simulink model "cartPend_HAC"  (R2023b)
settings: Solver=ode4  StartTime=0.0  StopTime=8  FixedStep=0.001  RelTol=1e-3
values from neighbouring files (symbols this model uses):
  alpha = 5/180*pi    (= 0.0872664625997)    [init_HAC_simulation.m]    (also in my_HAC_improved.m = params.alpha)
  beta = 50/180*pi    (= 0.872664625997)    [init_HAC_simulation.m]    (also in my_HAC_improved.m = params.beta)
  caseSwitch = 2    [init_HAC_simulation.m]
  E_up = m*g*L*cos(0)    [init_HAC_simulation.m]
  eta = 1.3    [init_HAC_simulation.m]
  Fc = 0.00040    (= 0.0004)    [init_HAC_simulation.m]
  g = 9.80665    [init_HAC_simulation.m]
  I = (1/3)*m*L^2    (= 0.0008739525)    [init_HAC_simulation.m]
  init_cont = [x_real(1),xd_real(1),q_real(1),qd_real(1)]    [RSHAC_real_data_processing.m]    (also in init_HAC_simulation.m = [0.1041, -0.2018, deg2rad(-14.9877), deg2rad(135.7108)])
  k_cw = 6    [init_HAC_simulation.m]
  k_em = 10    [init_HAC_simulation.m]
  k_lqr = discrete_lqr(m, M, L, I, g, kd, kt, Fc)    [init_HAC_simulation.m]
  k_su = 2    [init_HAC_simulation.m]
  k_vw = 2.5    [init_HAC_simulation.m]
  kd = 0.000161    [init_HAC_simulation.m]
  kdr = 0.000001    (= 1e-06)    [init_HAC_simulation.m]
  kt = 150    [init_HAC_simulation.m]
  L = 0.3/2    (= 0.15)    [init_HAC_simulation.m]
  m = 0.116527    [init_HAC_simulation.m]
  q_max = deg2rad(20)    [init_HAC_simulation.m]    (also in my_HAC_improved.m = X_max(3))
  q_min = -q_max    (= -0.261799387799)    [init_HAC_simulation.m]    (also in my_HAC_improved.m = X_min(3))
  q_sqm = zeros(1, n_rules_q)    [init_HAC_simulation.m]
  qd_max = 6    [init_HAC_simulation.m]    (also in my_HAC_improved.m = X_max(4))
  qd_min = -qd_max    (= -6)    [init_HAC_simulation.m]    (also in my_HAC_improved.m = X_min(4))
  qd_sqm = zeros(1, n_rules_qd)    [init_HAC_simulation.m]
  SQMs_state = zeros(1,n_rules)    [init_HAC_simulation.m]
  SQMs_u = zeros(1,n_rules)    [init_HAC_simulation.m]
  target_pos = 0    [init_HAC_simulation.m]
  u_max = 3 * g    (= 29.41995)    [init_HAC_simulation.m]    (also in my_HAC_improved.m = params.u_max)
  u_min = -u_max    (= -29.41995)    [init_HAC_simulation.m]    (also in my_HAC_improved.m = params.u_min)
  u_q_sqm = zeros(1, n_rules_q)    [init_HAC_simulation.m]
  u_qd_sqm = zeros(1, n_rules_qd)    [init_HAC_simulation.m]
  u_x_sqm = zeros(1, n_rules_x)    [init_HAC_simulation.m]
  u_xd_sqm = zeros(1, n_rules_xd)    [init_HAC_simulation.m]
  uMax = 3*g    (= 29.41995)    [init_HAC_simulation.m]
  w_high = 1    [init_HAC_simulation.m]    (also in my_HAC_improved.m = params.w_high)
  w_low = 0.25    [init_HAC_simulation.m]    (also in my_HAC_improved.m = params.w_low)
  x1_max = 0.43    [init_HAC_simulation.m]
  x2_max = 2    [init_HAC_simulation.m]
  x_max = 0.43    [init_HAC_simulation.m]    (also in my_HAC_improved.m = X_max(1))
  x_min = -x_max    (= -0.43)    [init_HAC_simulation.m]    (also in my_HAC_improved.m = X_min(1))
  x_sqm = zeros(1, n_rules_x)    [init_HAC_simulation.m]
  xd_max = 2.0    (= 2)    [init_HAC_simulation.m]    (also in my_HAC_improved.m = X_max(2))
  xd_min = -xd_max    (= -2)    [init_HAC_simulation.m]    (also in my_HAC_improved.m = X_min(2))
  xd_sqm = zeros(1, n_rules_xd)    [init_HAC_simulation.m]
undefined symbols (not defined in the file or in its folder): useThayLe
libraries: fuzblock x7, simulink x5, simulink_extras x2
settings Model: Creator=doann  LastModifiedBy=doann
settings OptimizationCC: ReuseModelBlockBuffer=off

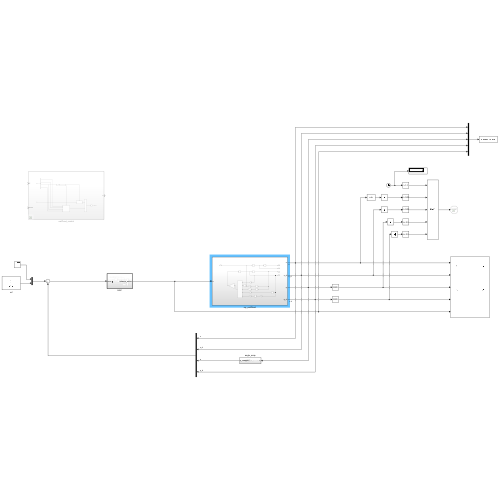
[thumbnail: Simulink's stored preview of the top-level diagram]
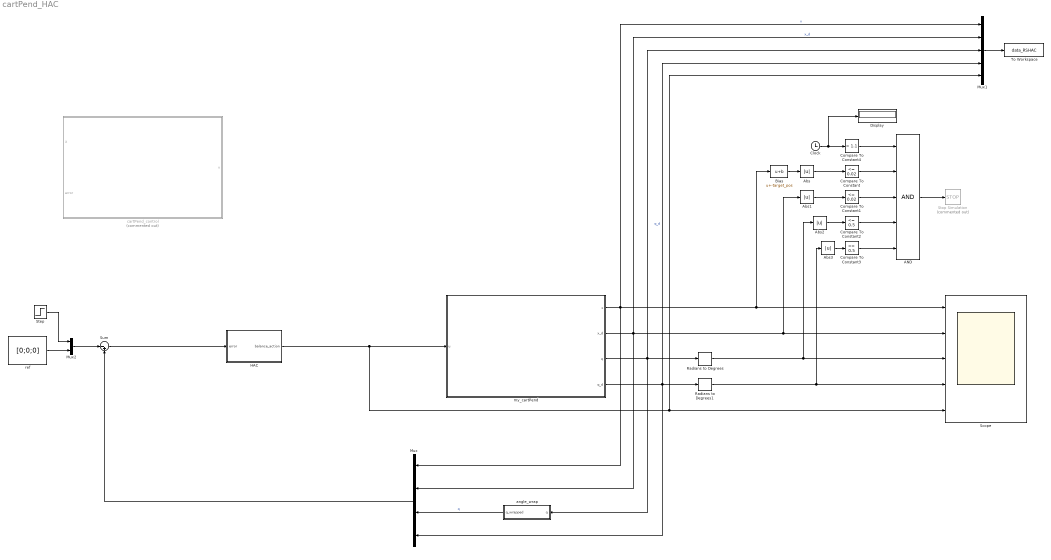
== system cartPend_HAC ==
  AND : Logic  Inputs=5  AllPortsSameDT=off  OutDataTypeStr=boolean
  Abs{,1..3} (4 alike) : Abs  SaturateOnIntegerOverflow=off
  Bias : Bias  Bias=-target_pos  SaturateOnIntegerOverflow=off
  Clock : Clock
  Compare To Constant : simulink/Logic and Bit Operations/Compare To Constant  relop=<=  const=0.02  OutDataTypeStr=boolean
  Compare To Constant1 : simulink/Logic and Bit Operations/Compare To Constant  relop=<=  const=0.02  OutDataTypeStr=boolean
  Compare To Constant2 : simulink/Logic and Bit Operations/Compare To Constant  relop=<=  const=0.5  OutDataTypeStr=boolean
  Compare To Constant3 : simulink/Logic and Bit Operations/Compare To Constant  relop=<=  const=0.5  OutDataTypeStr=boolean
  Compare To Constant4 : simulink/Logic and Bit Operations/Compare To Constant  relop=>  const=1.1  OutDataTypeStr=boolean
  Display : Display
  HAC : Subsystem  TreatAsAtomicUnit=on
  Mux : Mux
  Mux1 : Mux  Inputs=5
  Mux2 : Mux  Inputs=2
  Radians to Degrees : simulink_extras/Transformations/Radians to Degrees
  Radians to Degrees1 : simulink_extras/Transformations/Radians to Degrees
  Scope : Scope  NumInputPorts=5
  Step : Step  After=target_pos  SampleTime=0
  Stop Simulation : Stop  Commented=on
  Sum : Sum  Inputs=|-+
  To Workspace : ToWorkspace  VariableName=data_RSHAC  SaveFormat=Timeseries  SampleTime=-1
  angle_wrap : Subsystem
  cartPend_control : Subsystem  Commented=on  SystemSampleTime=0.001
  my_cartPend : Subsystem
  ref : Constant  Value=[0;0;0]  VectorParams1D=off
  wires:
  my_cartPend/1(x) -> Mux1/1, Bias/1, Scope/1, Mux/1  "x"
  my_cartPend/2(x_d) -> Mux1/2, Abs1/1, Scope/2, Mux/2  "x_d"
  Radians to Degrees/1 -> Abs2/1, Scope/3
  my_cartPend/4(q_d) -> Mux1/4, Radians to Degrees1/1, Mux/4  "q_d"
  Radians to Degrees1/1 -> Abs3/1, Scope/4
  my_cartPend/3(q) -> Mux1/3, Radians to Degrees/1, angle_wrap/1(q)
  angle_wrap/1(q_wrapped) -> Mux/3  "q"
  Mux/1 -> Sum/2
  Mux1/1 -> To Workspace/1
  Sum/1 -> HAC/1(error)
  HAC/1(balance_action) -> Mux1/5, Scope/5, my_cartPend/1(u)
  Compare To Constant/1 -> AND/2
  Compare To Constant1/1 -> AND/3
  Compare To Constant2/1 -> AND/4
  Compare To Constant3/1 -> AND/5
  Abs/1 -> Compare To Constant/1
  Abs1/1 -> Compare To Constant1/1
  Abs2/1 -> Compare To Constant2/1
  Abs3/1 -> Compare To Constant3/1
  Clock/1 -> Display/1, Compare To Constant4/1
  Compare To Constant4/1 -> AND/1
  Bias/1 -> Abs/1
  Step/1 -> Mux2/1
  ref/1 -> Mux2/2
  Mux2/1 -> Sum/1
  AND/1 -> Stop Simulation/1

== system cartPend_HAC/HAC ==
  error : Inport
  Constant : Constant  Value=caseSwitch
  Fuzzy_controller : Subsystem  TreatAsAtomicUnit=on
  HAC_thay_Le : Subsystem
  LQR : Subsystem
  Merge : Merge  Inputs=4
  RSHAC : Subsystem
  Switch Case : SwitchCase  CaseConditions={1,2,3,4}  ShowDefaultCase=off
  balance_action : Outport
  wires:
  error/1 -> HAC_thay_Le/1(error), RSHAC/1(error), Fuzzy_controller/1(error), LQR/1(error)
  Constant/1 -> Switch Case/1
  Switch Case/3 -> HAC_thay_Le/Action
  Switch Case/2 -> RSHAC/Action
  Switch Case/1 -> LQR/Action
  HAC_thay_Le/1(u) -> Merge/1
  RSHAC/1(u) -> Merge/2
  LQR/1(u) -> Merge/3
  Merge/1 -> balance_action/1
  Fuzzy_controller/1(u) -> Merge/4
  Switch Case/4 -> Fuzzy_controller/Action

== system cartPend_HAC/angle_wrap ==
  q : Inport
  Atan2 : Trigonometry  Operator=atan2
  Cos : Trigonometry  Operator=cos
  Sin : Trigonometry
  q_wrapped : Outport
  wires:
  Atan2/1 -> q_wrapped/1
  Sin/1 -> Atan2/1
  q/1 -> Cos/1, Sin/1
  Cos/1 -> Atan2/2

== system cartPend_HAC/cartPend_control ==
  X : Inport
  error : Inport  Port=2
  Abs : Abs  SaturateOnIntegerOverflow=off
  Demux : Demux
  HAC : Subsystem  TreatAsAtomicUnit=on
  If : If  IfExpression=u1 < angle_threshold
  Merge : Merge
  Saturation : Saturate  UpperLimit=uMax  LowerLimit=-uMax
  energy swing up : Subsystem  TreatAsAtomicUnit=on
  u : Outport
  wires:
  X/1 -> Demux/1
  Demux/3 -> Abs/1, energy swing up/3(x3)  "x3"
  Demux/4 -> energy swing up/4(x4)  "x4"
  Abs/1 -> If/1
  If/1 -> HAC/Action
  If/2 -> energy swing up/Action
  HAC/1(balance_action) -> Merge/1
  energy swing up/1(swing_up_action) -> Merge/2
  error/1 -> HAC/1(error)
  Demux/2 -> energy swing up/2(x2)  "x2"
  Demux/1 -> energy swing up/1(x1)  "x1"
  Merge/1 -> Saturation/1
  Saturation/1 -> u/1

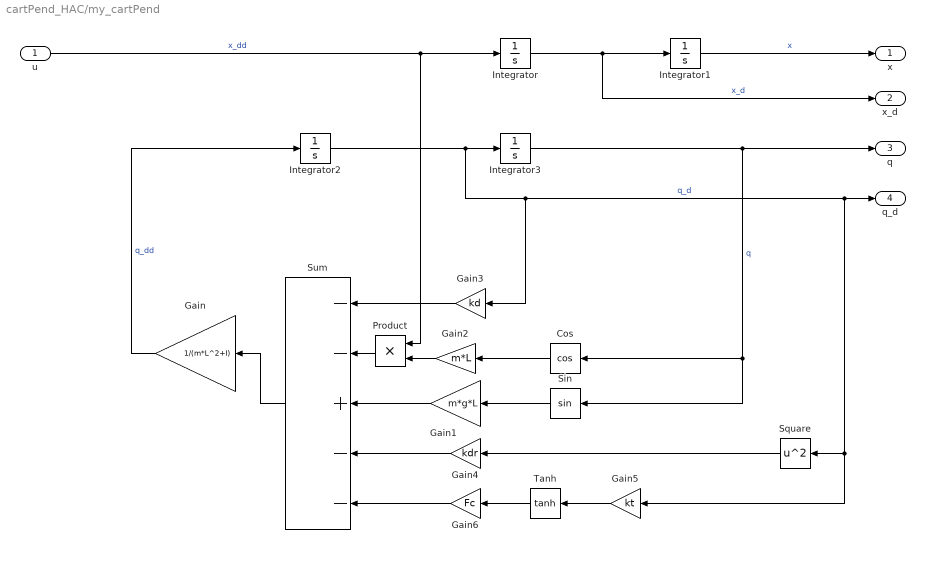
== system cartPend_HAC/my_cartPend ==
  u : Inport
  Cos : Trigonometry  Operator=cos
  Gain : Gain  Gain=1/(m*L^2+I)
  Gain1 : Gain  Gain=m*g*L
  Gain2 : Gain  Gain=m*L
  Gain3 : Gain  Gain=kd
  Gain4 : Gain  Gain=kdr
  Gain5 : Gain  Gain=kt
  Gain6 : Gain  Gain=Fc
  Integrator : Integrator  InitialCondition=init_cont(2)
  Integrator1 : Integrator  InitialCondition=init_cont(1)
  Integrator2 : Integrator  InitialCondition=init_cont(4)
  Integrator3 : Integrator  InitialCondition=init_cont(3)
  Product : Product
  Sin : Trigonometry
  Square : Math  Operator=square
  Sum : Sum  Inputs=--+--
  Tanh : Trigonometry  Operator=tanh
  x : Outport
  x_d : Outport  Port=2
  q : Outport  Port=3
  q_d : Outport  Port=4
  wires:
  Gain6/1 -> Sum/5
  Gain4/1 -> Sum/4
  Gain5/1 -> Tanh/1
  Tanh/1 -> Gain6/1
  Square/1 -> Gain4/1
  Product/1 -> Sum/2
  Gain2/1 -> Product/2
  Gain3/1 -> Sum/1
  Gain1/1 -> Sum/3
  Gain/1 -> Integrator2/1  "q_dd"
  Sum/1 -> Gain/1
  Cos/1 -> Gain2/1
  Sin/1 -> Gain1/1
  Integrator2/1 -> Integrator3/1, q_d/1, Square/1, Gain5/1, Gain3/1  "q_d"
  Integrator3/1 -> q/1, Cos/1, Sin/1  "q"
  Integrator1/1 -> x/1  "x"
  Integrator/1 -> Integrator1/1, x_d/1  "x_d"
  u/1 -> Integrator/1, Product/1  "x_dd"

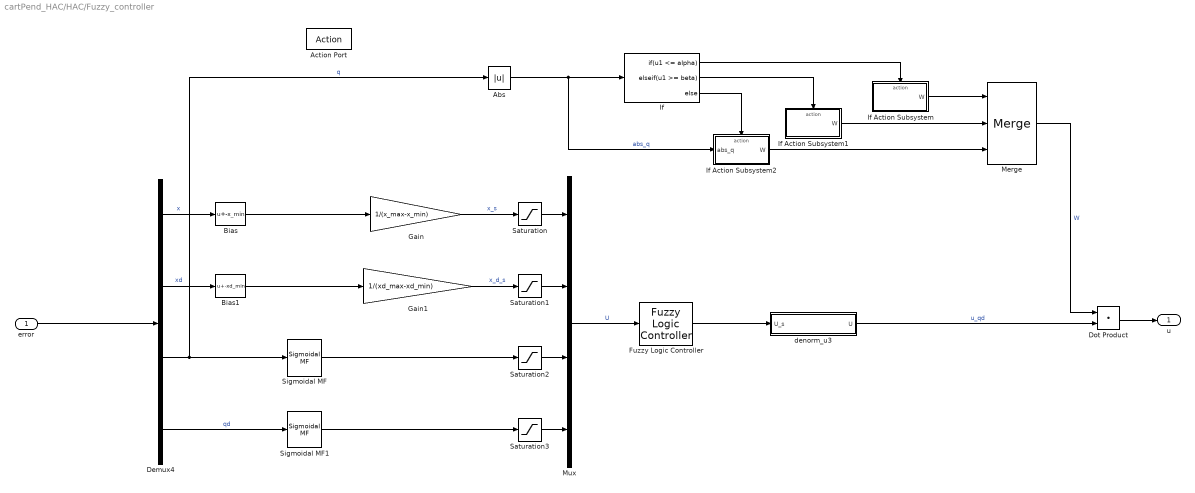
== system cartPend_HAC/HAC/Fuzzy_controller ==
  error : Inport
  Action Port : ActionPort  ActionPortLabel=case [ 4 ]:
  Abs : Abs  SaturateOnIntegerOverflow=off
  Bias : Bias  Bias=-x_min  SaturateOnIntegerOverflow=off
  Bias1 : Bias  Bias=-xd_min  SaturateOnIntegerOverflow=off
  Demux4 : Demux
  Dot Product : DotProduct  OutDataTypeStr=Inherit: Inherit via internal rule
  Fuzzy Logic Controller : fuzblock/Fuzzy Logic  Controller  FIS='fuzzy_ctrl_v2.fis'  OutputSampleNumber=101  DataType=double  FuzzifiedInputs=off  RuleFiringStrengths=off  RuleOutputs=off  AggregatedOutputs=off  SimulateUsing=Interpreted execution  OutOfRangeInputValueMessage=warning  NoRuleFiredMessage=warning  EmptyOutputFuzzySetMessage=warning
  Gain : Gain  Gain=1/(x_max-x_min)
  Gain1 : Gain  Gain=1/(xd_max-xd_min)
  If : If  IfExpression=u1 <= alpha  ElseIfExpressions=u1 >= beta
  If Action Subsystem : Subsystem  TreatAsAtomicUnit=on
  If Action Subsystem1 : Subsystem  TreatAsAtomicUnit=on
  If Action Subsystem2 : Subsystem  TreatAsAtomicUnit=on
  Merge : Merge  Inputs=3
  Mux : Mux
  Saturation{,1..3} (4 alike) : Saturate  UpperLimit=0.75  LowerLimit=0.25
  Sigmoidal MF : fuzblock/Membership  Functions/Sigmoidal MF  a=a_sigmoid_q  c=0
  Sigmoidal MF1 : fuzblock/Membership  Functions/Sigmoidal MF  a=a_sigmoid_q_d  c=0
  denorm_u3 : Subsystem
  u : Outport
  wires:
  Demux4/2 -> Bias1/1  "xd"
  Gain/1 -> Saturation/1  "x_s"
  Sigmoidal MF/1 -> Saturation2/1
  Demux4/4 -> Sigmoidal MF1/1  "qd"
  Bias/1 -> Gain/1
  Gain1/1 -> Saturation1/1  "x_d_s"
  Sigmoidal MF1/1 -> Saturation3/1
  Bias1/1 -> Gain1/1
  Demux4/1 -> Bias/1  "x"
  error/1 -> Demux4/1
  Mux/1 -> Fuzzy Logic Controller/1  "U"
  Fuzzy Logic Controller/1 -> denorm_u3/1(U_s)
  Saturation/1 -> Mux/1
  Saturation1/1 -> Mux/2
  Saturation2/1 -> Mux/3
  Saturation3/1 -> Mux/4
  If/2 -> If Action Subsystem1/Action
  If Action Subsystem2/1(W) -> Merge/3
  If/1 -> If Action Subsystem/Action
  If Action Subsystem1/1(W) -> Merge/2
  If/3 -> If Action Subsystem2/Action
  Demux4/3 -> Sigmoidal MF/1, Abs/1  "q"
  Abs/1 -> If Action Subsystem2/1(abs_q), If/1  "abs_q"
  If Action Subsystem/1(W) -> Merge/1
  Merge/1 -> Dot Product/1  "W"
  denorm_u3/1(U) -> Dot Product/2  "u_qd"
  Dot Product/1 -> u/1

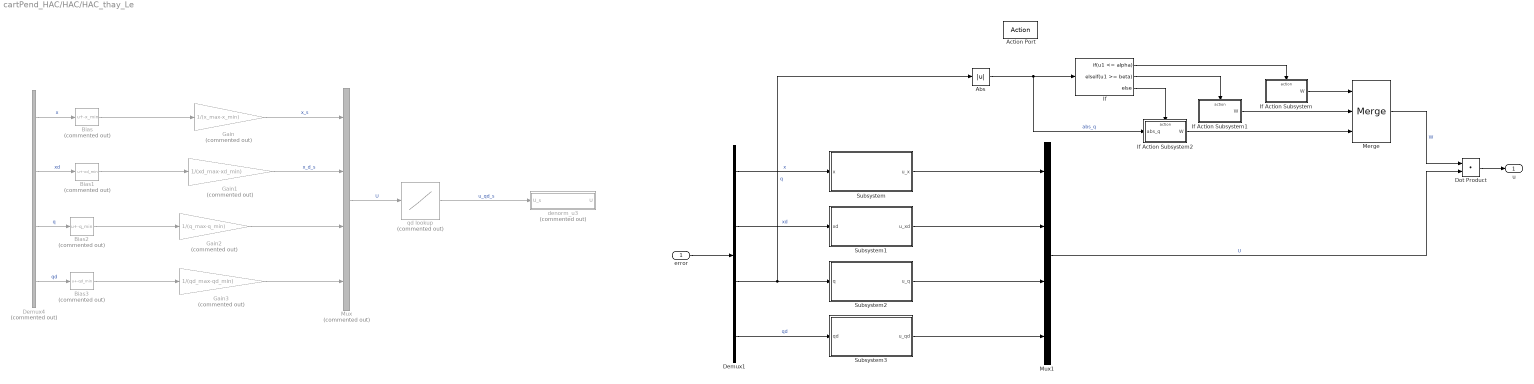
== system cartPend_HAC/HAC/HAC_thay_Le ==
  error : Inport
  Action Port : ActionPort  ActionPortLabel=case [ 3 ]:
  Abs : Abs  SaturateOnIntegerOverflow=off
  Bias : Bias  Commented=on  Bias=-x_min  SaturateOnIntegerOverflow=off
  Bias1 : Bias  Commented=on  Bias=-xd_min  SaturateOnIntegerOverflow=off
  Bias2 : Bias  Commented=on  Bias=-q_min  SaturateOnIntegerOverflow=off
  Bias3 : Bias  Commented=on  Bias=-qd_min  SaturateOnIntegerOverflow=off
  Demux1 : Demux
  Demux4 : Demux  Commented=on
  Dot Product : DotProduct  OutDataTypeStr=Inherit: Inherit via internal rule
  Gain : Gain  Commented=on  Gain=1/(x_max-x_min)
  Gain1 : Gain  Commented=on  Gain=1/(xd_max-xd_min)
  Gain2 : Gain  Commented=on  Gain=1/(q_max-q_min)
  Gain3 : Gain  Commented=on  Gain=1/(qd_max-qd_min)
  If : If  IfExpression=u1 <= alpha  ElseIfExpressions=u1 >= beta
  If Action Subsystem : Subsystem  TreatAsAtomicUnit=on
  If Action Subsystem1 : Subsystem  TreatAsAtomicUnit=on
  If Action Subsystem2 : Subsystem  TreatAsAtomicUnit=on
  Merge : Merge  Inputs=3
  Mux : Mux  Commented=on
  Mux1 : Mux
  Subsystem : Subsystem
  Subsystem1 : Subsystem
  Subsystem2 : Subsystem
  Subsystem3 : Subsystem
  denorm_u3 : Subsystem  Commented=on
  qd lookup : Lookup_n-D  Commented=on  NumberOfTableDimensions=1  BreakpointsForDimension1=SQMs_state  Table=SQMs_u  InternalRulePriority=Speed  RndMeth=Simplest
  u : Outport
  wires:
  Merge/1 -> Dot Product/1  "W"
  Demux4/4 -> Bias3/1  "qd"
  qd lookup/1 -> denorm_u3/1(U_s)  "u_qd_s"
  Bias3/1 -> Gain3/1
  Bias2/1 -> Gain2/1
  Demux4/2 -> Bias1/1  "xd"
  Bias1/1 -> Gain1/1
  Demux4/1 -> Bias/1  "x"
  Bias/1 -> Gain/1
  Dot Product/1 -> u/1
  If Action Subsystem2/1(W) -> Merge/3
  If Action Subsystem1/1(W) -> Merge/2
  If Action Subsystem/1(W) -> Merge/1
  If/3 -> If Action Subsystem2/Action
  If/2 -> If Action Subsystem1/Action
  If/1 -> If Action Subsystem/Action
  Abs/1 -> If Action Subsystem2/1(abs_q), If/1  "abs_q"
  Demux4/3 -> Bias2/1  "q"
  Gain1/1 -> Mux/2  "x_d_s"
  Gain/1 -> Mux/1  "x_s"
  Gain2/1 -> Mux/3
  Gain3/1 -> Mux/4
  Mux/1 -> qd lookup/1  "U"
  Demux1/1 -> Subsystem/1(x)  "x"
  Subsystem/1(u_x) -> Mux1/1
  Demux1/2 -> Subsystem1/1(xd)  "xd"
  Subsystem1/1(u_xd) -> Mux1/2
  Demux1/3 -> Abs/1, Subsystem2/1(q)  "q"
  Subsystem2/1(u_q) -> Mux1/3
  Demux1/4 -> Subsystem3/1(qd)  "qd"
  Subsystem3/1(u_qd) -> Mux1/4
  error/1 -> Demux1/1
  Mux1/1 -> Dot Product/2  "U"

== system cartPend_HAC/HAC/LQR ==
  error : Inport
  Action Port : ActionPort  ActionPortLabel=case [ 1 ]:
  Gain : Gain  Gain=k_lqr  Multiplication=Matrix(K*u)
  Gain1 : Gain  Gain=-1
  u : Outport
  wires:
  Gain1/1 -> Gain/1
  Gain/1 -> u/1
  error/1 -> Gain1/1

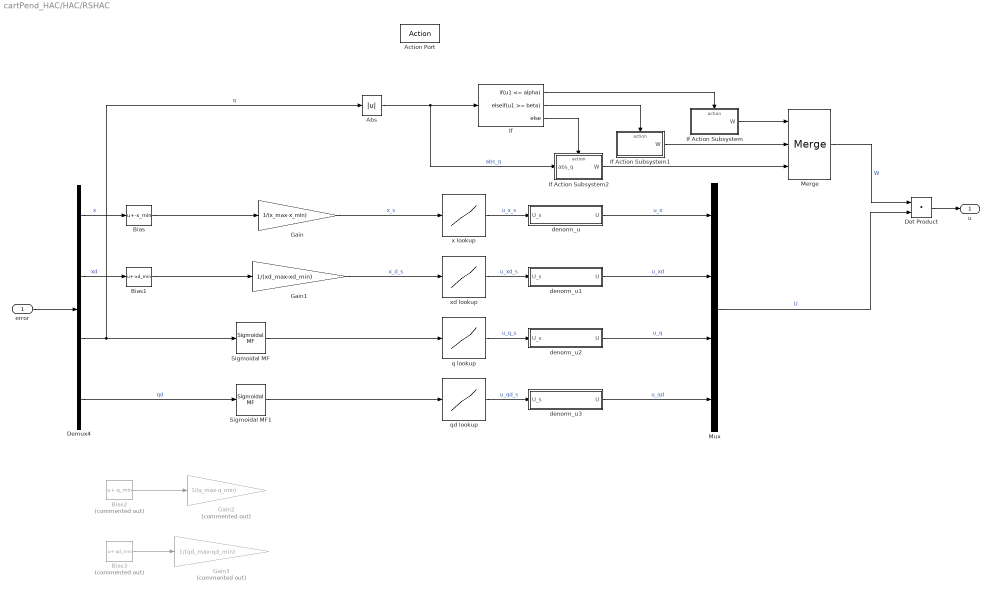
== system cartPend_HAC/HAC/RSHAC ==
  error : Inport
  Action Port : ActionPort  ActionPortLabel=case [ 2 ]:
  Abs : Abs  SaturateOnIntegerOverflow=off
  Bias : Bias  Bias=-x_min  SaturateOnIntegerOverflow=off
  Bias1 : Bias  Bias=-xd_min  SaturateOnIntegerOverflow=off
  Bias2 : Bias  Commented=on  Bias=-q_min  SaturateOnIntegerOverflow=off
  Bias3 : Bias  Commented=on  Bias=-qd_min  SaturateOnIntegerOverflow=off
  Demux4 : Demux
  Dot Product : DotProduct  OutDataTypeStr=Inherit: Inherit via internal rule
  Gain : Gain  Gain=1/(x_max-x_min)
  Gain1 : Gain  Gain=1/(xd_max-xd_min)
  Gain2 : Gain  Commented=on  Gain=1/(q_max-q_min)
  Gain3 : Gain  Commented=on  Gain=1/(qd_max-qd_min)
  If : If  IfExpression=u1 <= alpha  ElseIfExpressions=u1 >= beta
  If Action Subsystem : Subsystem  TreatAsAtomicUnit=on
  If Action Subsystem1 : Subsystem  TreatAsAtomicUnit=on
  If Action Subsystem2 : Subsystem  TreatAsAtomicUnit=on
  Merge : Merge  Inputs=3
  Mux : Mux
  Sigmoidal MF : fuzblock/Membership  Functions/Sigmoidal MF  a=a_sigmoid_q  c=0
  Sigmoidal MF1 : fuzblock/Membership  Functions/Sigmoidal MF  a=a_sigmoid_q_d  c=0
  denorm_u : Subsystem
  denorm_u1 : Subsystem
  denorm_u2 : Subsystem
  denorm_u3 : Subsystem
  q lookup : Lookup_n-D  NumberOfTableDimensions=1  BreakpointsForDimension1=q_sqm  Table=u_q_sqm  InternalRulePriority=Speed  RndMeth=Simplest
  qd lookup : Lookup_n-D  NumberOfTableDimensions=1  BreakpointsForDimension1=qd_sqm  Table=u_qd_sqm  InternalRulePriority=Speed  RndMeth=Simplest
  x lookup : Lookup_n-D  NumberOfTableDimensions=1  BreakpointsForDimension1=x_sqm  Table=u_x_sqm  InternalRulePriority=Speed  RndMeth=Simplest
  xd lookup : Lookup_n-D  NumberOfTableDimensions=1  BreakpointsForDimension1=xd_sqm  Table=u_xd_sqm  InternalRulePriority=Speed  RndMeth=Simplest
  u : Outport
  wires:
  Demux4/3 -> Sigmoidal MF/1, Abs/1  "q"
  Gain/1 -> x lookup/1  "x_s"
  Abs/1 -> If Action Subsystem2/1(abs_q), If/1  "abs_q"
  If/1 -> If Action Subsystem/Action
  If/2 -> If Action Subsystem1/Action
  If/3 -> If Action Subsystem2/Action
  If Action Subsystem/1(W) -> Merge/1
  If Action Subsystem1/1(W) -> Merge/2
  If Action Subsystem2/1(W) -> Merge/3
  Dot Product/1 -> u/1
  error/1 -> Demux4/1
  Bias/1 -> Gain/1
  Demux4/1 -> Bias/1  "x"
  Bias1/1 -> Gain1/1
  Gain1/1 -> xd lookup/1  "x_d_s"
  Demux4/2 -> Bias1/1  "xd"
  Bias2/1 -> Gain2/1
  Bias3/1 -> Gain3/1
  x lookup/1 -> denorm_u/1(U_s)  "u_x_s"
  denorm_u/1(U) -> Mux/1  "u_x"
  xd lookup/1 -> denorm_u1/1(U_s)  "u_xd_s"
  denorm_u1/1(U) -> Mux/2  "u_xd"
  q lookup/1 -> denorm_u2/1(U_s)  "u_q_s"
  denorm_u2/1(U) -> Mux/3  "u_q"
  qd lookup/1 -> denorm_u3/1(U_s)  "u_qd_s"
  denorm_u3/1(U) -> Mux/4  "u_qd"
  Mux/1 -> Dot Product/2  "U"
  Sigmoidal MF/1 -> q lookup/1
  Sigmoidal MF1/1 -> qd lookup/1
  Demux4/4 -> Sigmoidal MF1/1  "qd"
  Merge/1 -> Dot Product/1  "W"

== system cartPend_HAC/cartPend_control/HAC ==
  error : Inport
  Action Port : ActionPort  ActionPortLabel=if(u1 < angle_threshold)
  Constant : Constant  Value=useThayLe
  HAC : Subsystem
  HAC_thay_Le : Subsystem
  Switch : Switch  Criteria=u2 ~= 0  SaturateOnIntegerOverflow=off  InputSameDT=off
  balance_action : Outport
  wires:
  Constant/1 -> Switch/2
  HAC_thay_Le/1(u) -> Switch/1
  HAC/1(u) -> Switch/3
  Switch/1 -> balance_action/1
  error/1 -> HAC/1(error), HAC_thay_Le/1(error)

== system cartPend_HAC/cartPend_control/energy swing up ==
  x1 : Inport
  x2 : Inport  Port=2
  x3 : Inport  Port=3
  x4 : Inport  Port=4
  Action Port : ActionPort  ActionPortLabel=else
  Sum : Sum  Inputs=++++
  energy injection : Subsystem
  energy maintenance : Subsystem
  position potential well : Subsystem
  velocity potential well : Subsystem
  swing_up_action : Outport
  wires:
  energy injection/1(u_su) -> Sum/3
  x2/1 -> velocity potential well/1(x2)  "x2"
  velocity potential well/1(u_vw) -> Sum/2
  Sum/1 -> swing_up_action/1
  energy maintenance/1(u_em) -> Sum/4
  x3/1 -> energy maintenance/1(x3), energy injection/1(x3)  "x3"
  x1/1 -> position potential well/1(x1)  "x1"
  x4/1 -> energy injection/2(x4), energy maintenance/2(x4)  "x4"
  position potential well/1(u_cw) -> Sum/1

== system cartPend_HAC/HAC/Fuzzy_controller/If Action Subsystem ==
  Action Port : ActionPort  ActionPortLabel=if(u1 <= alpha)
  weight : Constant  Value=[0.25; 0.25; 0.25; 0.25]  VectorParams1D=off
  W : Outport
  wires:
  weight/1 -> W/1

== system cartPend_HAC/HAC/Fuzzy_controller/If Action Subsystem1 ==
  Action Port : ActionPort  ActionPortLabel=elseif(u1 >= beta)
  weights : Constant  Value=[0; 0; 1; 0]  VectorParams1D=off
  W : Outport
  wires:
  weights/1 -> W/1

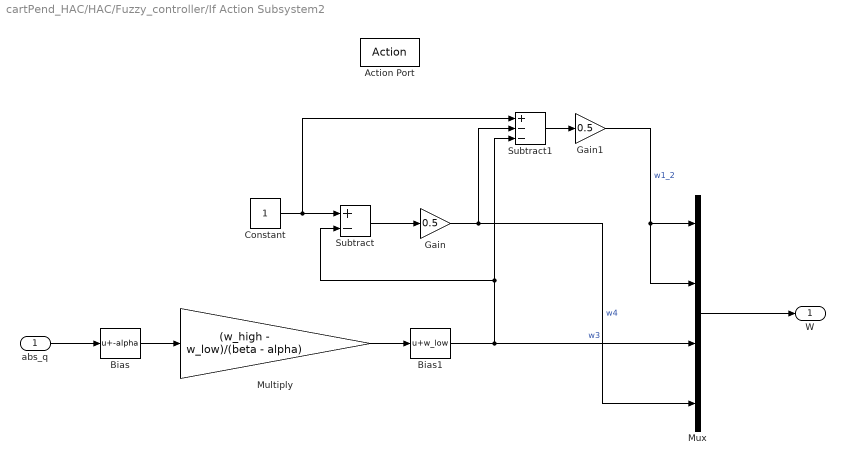
== system cartPend_HAC/HAC/Fuzzy_controller/If Action Subsystem2 ==
  abs_q : Inport
  Action Port : ActionPort  ActionPortLabel=else
  Bias : Bias  Bias=-alpha  SaturateOnIntegerOverflow=off
  Bias1 : Bias  Bias=w_low  SaturateOnIntegerOverflow=off
  Constant : Constant
  Gain : Gain  Gain=0.5
  Gain1 : Gain  Gain=0.5
  Multiply : Gain  Gain=(w_high - w_low)/(beta - alpha)
  Mux : Mux
  Subtract : Sum  Inputs=+-
  Subtract1 : Sum  Inputs=+--
  W : Outport
  wires:
  Mux/1 -> W/1
  abs_q/1 -> Bias/1
  Bias/1 -> Multiply/1
  Multiply/1 -> Bias1/1
  Bias1/1 -> Subtract/2, Subtract1/3, Mux/3  "w3"
  Constant/1 -> Subtract1/1, Subtract/1
  Subtract/1 -> Gain/1
  Gain/1 -> Subtract1/2, Mux/4  "w4"
  Subtract1/1 -> Gain1/1
  Gain1/1 -> Mux/1, Mux/2  "w1_2"

== system cartPend_HAC/HAC/Fuzzy_controller/denorm_u3 ==
  U_s : Inport
  Bias : Bias  Bias=2*u_min  SaturateOnIntegerOverflow=off
  Gain : Gain  Gain=4*u_max
  U : Outport
  wires:
  U_s/1 -> Gain/1
  Gain/1 -> Bias/1
  Bias/1 -> U/1

== system cartPend_HAC/HAC/HAC_thay_Le/If Action Subsystem ==
  Action Port : ActionPort  ActionPortLabel=if(u1 <= alpha)
  weight : Constant  Value=[0.25; 0.25; 0.25; 0.25]  VectorParams1D=off
  W : Outport
  wires:
  weight/1 -> W/1

== system cartPend_HAC/HAC/HAC_thay_Le/If Action Subsystem1 ==
  Action Port : ActionPort  ActionPortLabel=elseif(u1 >= beta)
  weights : Constant  Value=[0; 0; 1; 0]  VectorParams1D=off
  W : Outport
  wires:
  weights/1 -> W/1

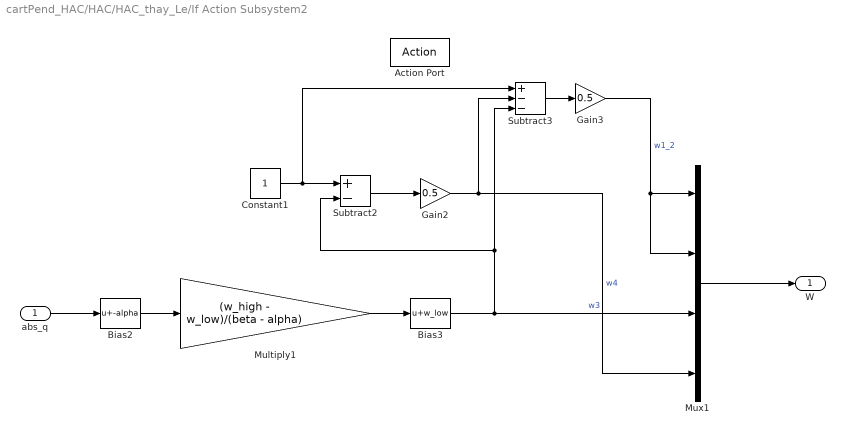
== system cartPend_HAC/HAC/HAC_thay_Le/If Action Subsystem2 ==
  abs_q : Inport
  Action Port : ActionPort  ActionPortLabel=else
  Bias2 : Bias  Bias=-alpha  SaturateOnIntegerOverflow=off
  Bias3 : Bias  Bias=w_low  SaturateOnIntegerOverflow=off
  Constant1 : Constant
  Gain2 : Gain  Gain=0.5
  Gain3 : Gain  Gain=0.5
  Multiply1 : Gain  Gain=(w_high - w_low)/(beta - alpha)
  Mux1 : Mux
  Subtract2 : Sum  Inputs=+-
  Subtract3 : Sum  Inputs=+--
  W : Outport
  wires:
  Subtract3/1 -> Gain3/1
  Gain2/1 -> Subtract3/2, Mux1/4  "w4"
  Bias3/1 -> Subtract2/2, Subtract3/3, Mux1/3  "w3"
  Bias2/1 -> Multiply1/1
  Gain3/1 -> Mux1/1, Mux1/2  "w1_2"
  Subtract2/1 -> Gain2/1
  Multiply1/1 -> Bias3/1
  Constant1/1 -> Subtract3/1, Subtract2/1
  Mux1/1 -> W/1
  abs_q/1 -> Bias2/1

== system cartPend_HAC/HAC/HAC_thay_Le/Subsystem ==
  x : Inport
  If Action Subsystem3 : Subsystem  TreatAsAtomicUnit=on
  If Action Subsystem4 : Subsystem  TreatAsAtomicUnit=on
  If Action Subsystem5 : Subsystem  TreatAsAtomicUnit=on
  If1 : If  IfExpression=u1 <= x_min  ElseIfExpressions=u1 >= x_max
  Merge1 : Merge  Inputs=3
  u_x : Outport
  wires:
  If1/1 -> If Action Subsystem3/Action
  If Action Subsystem3/1(u_min) -> Merge1/1
  Merge1/1 -> u_x/1
  x/1 -> If Action Subsystem5/1(x), If1/1
  If1/3 -> If Action Subsystem5/Action
  If1/2 -> If Action Subsystem4/Action
  If Action Subsystem5/1(u_x) -> Merge1/3
  If Action Subsystem4/1(u_max) -> Merge1/2

== system cartPend_HAC/HAC/HAC_thay_Le/Subsystem1 ==
  xd : Inport
  If Action Subsystem3 : Subsystem  TreatAsAtomicUnit=on
  If Action Subsystem4 : Subsystem  TreatAsAtomicUnit=on
  If Action Subsystem5 : Subsystem  TreatAsAtomicUnit=on
  If1 : If  IfExpression=u1 <= xd_min  ElseIfExpressions=u1 >= xd_max
  Merge1 : Merge  Inputs=3
  u_xd : Outport
  wires:
  If Action Subsystem4/1(u_max) -> Merge1/2
  If Action Subsystem5/1(u_xd) -> Merge1/3
  If1/2 -> If Action Subsystem4/Action
  If1/3 -> If Action Subsystem5/Action
  xd/1 -> If1/1, If Action Subsystem5/1(xd)
  Merge1/1 -> u_xd/1
  If Action Subsystem3/1(u_min) -> Merge1/1
  If1/1 -> If Action Subsystem3/Action

== system cartPend_HAC/HAC/HAC_thay_Le/Subsystem2 ==
  q : Inport
  If Action Subsystem3 : Subsystem  TreatAsAtomicUnit=on
  If Action Subsystem4 : Subsystem  TreatAsAtomicUnit=on
  If Action Subsystem5 : Subsystem  TreatAsAtomicUnit=on
  If1 : If  IfExpression=u1 <= q_min  ElseIfExpressions=u1 >= q_max
  Merge1 : Merge  Inputs=3
  u_q : Outport
  wires:
  If1/1 -> If Action Subsystem3/Action
  If Action Subsystem3/1(u_min) -> Merge1/1
  Merge1/1 -> u_q/1
  q/1 -> If Action Subsystem5/1(q), If1/1
  If1/3 -> If Action Subsystem5/Action
  If1/2 -> If Action Subsystem4/Action
  If Action Subsystem5/1(u_q) -> Merge1/3
  If Action Subsystem4/1(u_max) -> Merge1/2

== system cartPend_HAC/HAC/HAC_thay_Le/Subsystem3 ==
  qd : Inport
  If Action Subsystem3 : Subsystem  TreatAsAtomicUnit=on
  If Action Subsystem4 : Subsystem  TreatAsAtomicUnit=on
  If Action Subsystem5 : Subsystem  TreatAsAtomicUnit=on
  If1 : If  IfExpression=u1 <= qd_min  ElseIfExpressions=u1 >= qd_max
  Merge1 : Merge  Inputs=3
  u_qd : Outport
  wires:
  If Action Subsystem4/1(u_max) -> Merge1/2
  If Action Subsystem5/1(u_qd) -> Merge1/3
  If1/2 -> If Action Subsystem4/Action
  If1/3 -> If Action Subsystem5/Action
  qd/1 -> If1/1, If Action Subsystem5/1(qd)
  Merge1/1 -> u_qd/1
  If Action Subsystem3/1(u_min) -> Merge1/1
  If1/1 -> If Action Subsystem3/Action

== system cartPend_HAC/HAC/HAC_thay_Le/denorm_u3 ==
  U_s : Inport
  Bias : Bias  Bias=u_min  SaturateOnIntegerOverflow=off
  Gain : Gain  Gain=u_max - u_min
  U : Outport
  wires:
  U_s/1 -> Gain/1
  Gain/1 -> Bias/1
  Bias/1 -> U/1

== system cartPend_HAC/HAC/RSHAC/If Action Subsystem ==
  Action Port : ActionPort  ActionPortLabel=if(u1 <= alpha)
  weight : Constant  Value=[0.25; 0.25; 0.25; 0.25]  VectorParams1D=off
  W : Outport
  wires:
  weight/1 -> W/1

== system cartPend_HAC/HAC/RSHAC/If Action Subsystem1 ==
  Action Port : ActionPort  ActionPortLabel=elseif(u1 >= beta)
  weights : Constant  Value=[0; 0; 1; 0]  VectorParams1D=off
  W : Outport
  wires:
  weights/1 -> W/1

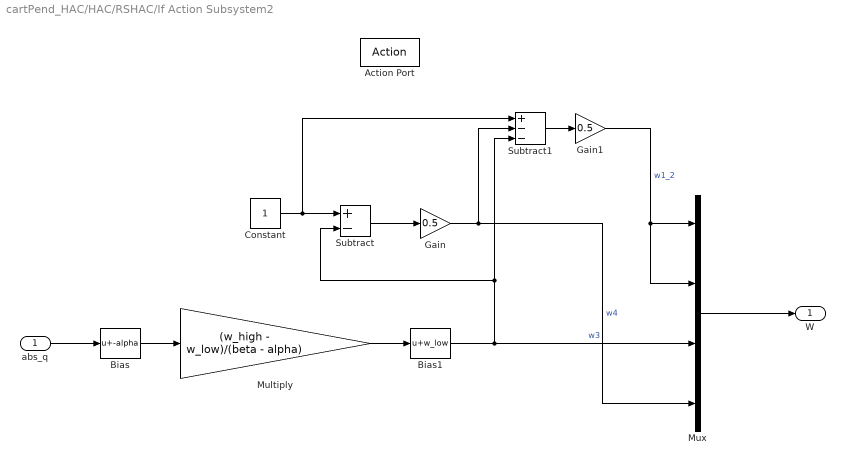
== system cartPend_HAC/HAC/RSHAC/If Action Subsystem2 ==
  abs_q : Inport
  Action Port : ActionPort  ActionPortLabel=else
  Bias : Bias  Bias=-alpha  SaturateOnIntegerOverflow=off
  Bias1 : Bias  Bias=w_low  SaturateOnIntegerOverflow=off
  Constant : Constant
  Gain : Gain  Gain=0.5
  Gain1 : Gain  Gain=0.5
  Multiply : Gain  Gain=(w_high - w_low)/(beta - alpha)
  Mux : Mux
  Subtract : Sum  Inputs=+-
  Subtract1 : Sum  Inputs=+--
  W : Outport
  wires:
  Mux/1 -> W/1
  abs_q/1 -> Bias/1
  Bias/1 -> Multiply/1
  Multiply/1 -> Bias1/1
  Bias1/1 -> Subtract/2, Subtract1/3, Mux/3  "w3"
  Constant/1 -> Subtract1/1, Subtract/1
  Subtract/1 -> Gain/1
  Gain/1 -> Subtract1/2, Mux/4  "w4"
  Subtract1/1 -> Gain1/1
  Gain1/1 -> Mux/1, Mux/2  "w1_2"

== system cartPend_HAC/HAC/RSHAC/denorm_u ==
  U_s : Inport
  Bias : Bias  Bias=u_min  SaturateOnIntegerOverflow=off
  Gain : Gain  Gain=u_max - u_min
  U : Outport
  wires:
  U_s/1 -> Gain/1
  Gain/1 -> Bias/1
  Bias/1 -> U/1

== system cartPend_HAC/HAC/RSHAC/denorm_u1 ==
  U_s : Inport
  Bias : Bias  Bias=u_min  SaturateOnIntegerOverflow=off
  Gain : Gain  Gain=u_max - u_min
  U : Outport
  wires:
  Bias/1 -> U/1
  Gain/1 -> Bias/1
  U_s/1 -> Gain/1

== system cartPend_HAC/HAC/RSHAC/denorm_u2 ==
  U_s : Inport
  Bias : Bias  Bias=u_min  SaturateOnIntegerOverflow=off
  Gain : Gain  Gain=u_max - u_min
  U : Outport
  wires:
  U_s/1 -> Gain/1
  Gain/1 -> Bias/1
  Bias/1 -> U/1

== system cartPend_HAC/HAC/RSHAC/denorm_u3 ==
  U_s : Inport
  Bias : Bias  Bias=u_min  SaturateOnIntegerOverflow=off
  Gain : Gain  Gain=u_max - u_min
  U : Outport
  wires:
  Bias/1 -> U/1
  Gain/1 -> Bias/1
  U_s/1 -> Gain/1

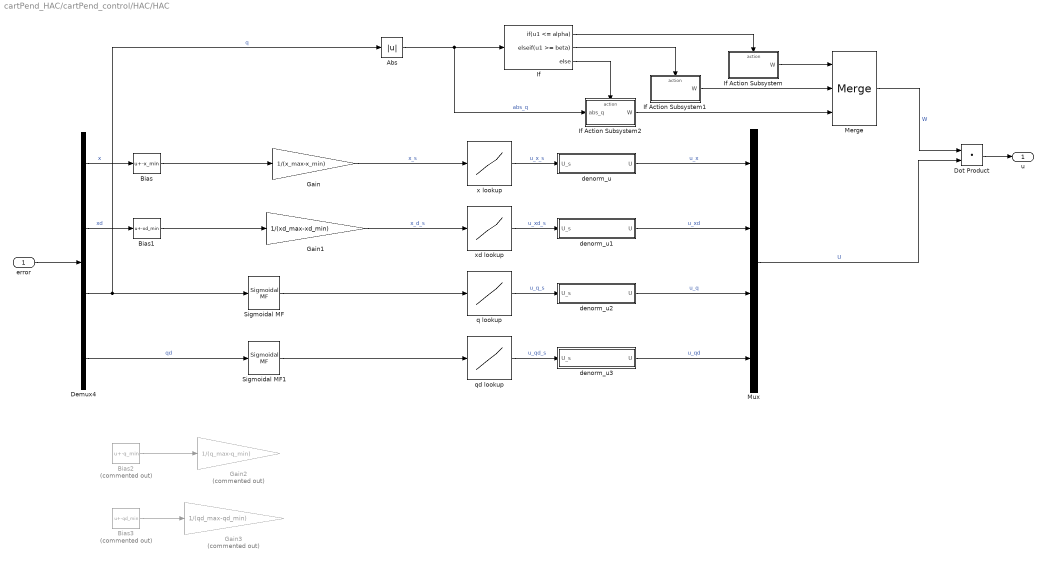
== system cartPend_HAC/cartPend_control/HAC/HAC ==
  error : Inport
  Abs : Abs  SaturateOnIntegerOverflow=off
  Bias : Bias  Bias=-x_min  SaturateOnIntegerOverflow=off
  Bias1 : Bias  Bias=-xd_min  SaturateOnIntegerOverflow=off
  Bias2 : Bias  Commented=on  Bias=-q_min  SaturateOnIntegerOverflow=off
  Bias3 : Bias  Commented=on  Bias=-qd_min  SaturateOnIntegerOverflow=off
  Demux4 : Demux
  Dot Product : DotProduct  OutDataTypeStr=Inherit: Inherit via internal rule
  Gain : Gain  Gain=1/(x_max-x_min)
  Gain1 : Gain  Gain=1/(xd_max-xd_min)
  Gain2 : Gain  Commented=on  Gain=1/(q_max-q_min)
  Gain3 : Gain  Commented=on  Gain=1/(qd_max-qd_min)
  If : If  IfExpression=u1 <= alpha  ElseIfExpressions=u1 >= beta
  If Action Subsystem : Subsystem  TreatAsAtomicUnit=on
  If Action Subsystem1 : Subsystem  TreatAsAtomicUnit=on
  If Action Subsystem2 : Subsystem  TreatAsAtomicUnit=on
  Merge : Merge  Inputs=3
  Mux : Mux
  Sigmoidal MF : fuzblock/Membership  Functions/Sigmoidal MF  a=a_sigmoid_q  c=0
  Sigmoidal MF1 : fuzblock/Membership  Functions/Sigmoidal MF  a=a_sigmoid_q_d  c=0
  denorm_u : Subsystem
  denorm_u1 : Subsystem
  denorm_u2 : Subsystem
  denorm_u3 : Subsystem
  q lookup : Lookup_n-D  NumberOfTableDimensions=1  BreakpointsForDimension1=q_sqm  Table=u_q_sqm  InternalRulePriority=Speed  RndMeth=Simplest
  qd lookup : Lookup_n-D  NumberOfTableDimensions=1  BreakpointsForDimension1=qd_sqm  Table=u_qd_sqm  InternalRulePriority=Speed  RndMeth=Simplest
  x lookup : Lookup_n-D  NumberOfTableDimensions=1  BreakpointsForDimension1=x_sqm  Table=u_x_sqm  InternalRulePriority=Speed  RndMeth=Simplest
  xd lookup : Lookup_n-D  NumberOfTableDimensions=1  BreakpointsForDimension1=xd_sqm  Table=u_xd_sqm  InternalRulePriority=Speed  RndMeth=Simplest
  u : Outport
  wires:
  Demux4/3 -> Sigmoidal MF/1, Abs/1  "q"
  Gain/1 -> x lookup/1  "x_s"
  Abs/1 -> If Action Subsystem2/1(abs_q), If/1  "abs_q"
  If/1 -> If Action Subsystem/Action
  If/2 -> If Action Subsystem1/Action
  If/3 -> If Action Subsystem2/Action
  If Action Subsystem/1(W) -> Merge/1
  If Action Subsystem1/1(W) -> Merge/2
  If Action Subsystem2/1(W) -> Merge/3
  Dot Product/1 -> u/1
  error/1 -> Demux4/1
  Bias/1 -> Gain/1
  Demux4/1 -> Bias/1  "x"
  Bias1/1 -> Gain1/1
  Gain1/1 -> xd lookup/1  "x_d_s"
  Demux4/2 -> Bias1/1  "xd"
  Bias2/1 -> Gain2/1
  Bias3/1 -> Gain3/1
  x lookup/1 -> denorm_u/1(U_s)  "u_x_s"
  denorm_u/1(U) -> Mux/1  "u_x"
  xd lookup/1 -> denorm_u1/1(U_s)  "u_xd_s"
  denorm_u1/1(U) -> Mux/2  "u_xd"
  q lookup/1 -> denorm_u2/1(U_s)  "u_q_s"
  denorm_u2/1(U) -> Mux/3  "u_q"
  qd lookup/1 -> denorm_u3/1(U_s)  "u_qd_s"
  denorm_u3/1(U) -> Mux/4  "u_qd"
  Mux/1 -> Dot Product/2  "U"
  Sigmoidal MF/1 -> q lookup/1
  Sigmoidal MF1/1 -> qd lookup/1
  Demux4/4 -> Sigmoidal MF1/1  "qd"
  Merge/1 -> Dot Product/1  "W"

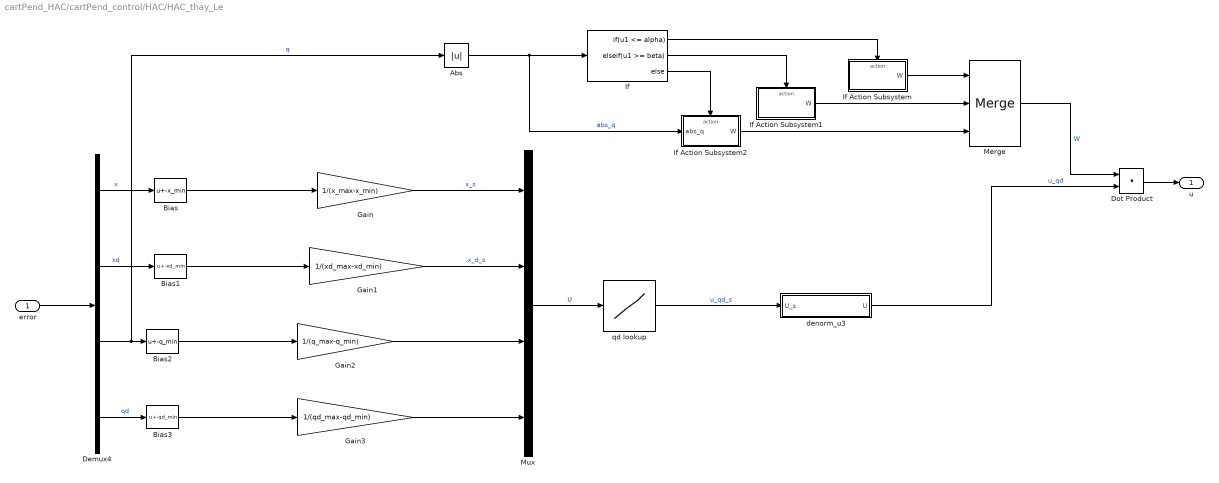
== system cartPend_HAC/cartPend_control/HAC/HAC_thay_Le ==
  error : Inport
  Abs : Abs  SaturateOnIntegerOverflow=off
  Bias : Bias  Bias=-x_min  SaturateOnIntegerOverflow=off
  Bias1 : Bias  Bias=-xd_min  SaturateOnIntegerOverflow=off
  Bias2 : Bias  Bias=-q_min  SaturateOnIntegerOverflow=off
  Bias3 : Bias  Bias=-qd_min  SaturateOnIntegerOverflow=off
  Demux4 : Demux
  Dot Product : DotProduct  OutDataTypeStr=Inherit: Inherit via internal rule
  Gain : Gain  Gain=1/(x_max-x_min)
  Gain1 : Gain  Gain=1/(xd_max-xd_min)
  Gain2 : Gain  Gain=1/(q_max-q_min)
  Gain3 : Gain  Gain=1/(qd_max-qd_min)
  If : If  IfExpression=u1 <= alpha  ElseIfExpressions=u1 >= beta
  If Action Subsystem : Subsystem  TreatAsAtomicUnit=on
  If Action Subsystem1 : Subsystem  TreatAsAtomicUnit=on
  If Action Subsystem2 : Subsystem  TreatAsAtomicUnit=on
  Merge : Merge  Inputs=3
  Mux : Mux
  denorm_u3 : Subsystem
  qd lookup : Lookup_n-D  NumberOfTableDimensions=1  BreakpointsForDimension1=[0.25, 0.5, 0.75]  Table=[0.25, 0.5, 0.75]  InternalRulePriority=Speed  RndMeth=Simplest
  u : Outport
  wires:
  Merge/1 -> Dot Product/1  "W"
  Demux4/4 -> Bias3/1  "qd"
  qd lookup/1 -> denorm_u3/1(U_s)  "u_qd_s"
  Bias3/1 -> Gain3/1
  Bias2/1 -> Gain2/1
  Demux4/2 -> Bias1/1  "xd"
  Bias1/1 -> Gain1/1
  Demux4/1 -> Bias/1  "x"
  Bias/1 -> Gain/1
  error/1 -> Demux4/1
  Dot Product/1 -> u/1
  If Action Subsystem2/1(W) -> Merge/3
  If Action Subsystem1/1(W) -> Merge/2
  If Action Subsystem/1(W) -> Merge/1
  If/3 -> If Action Subsystem2/Action
  If/2 -> If Action Subsystem1/Action
  If/1 -> If Action Subsystem/Action
  Abs/1 -> If/1, If Action Subsystem2/1(abs_q)  "abs_q"
  Demux4/3 -> Bias2/1, Abs/1  "q"
  Gain1/1 -> Mux/2  "x_d_s"
  Gain/1 -> Mux/1  "x_s"
  Gain2/1 -> Mux/3
  Gain3/1 -> Mux/4
  Mux/1 -> qd lookup/1  "U"
  denorm_u3/1(U) -> Dot Product/2  "u_qd"

== system cartPend_HAC/cartPend_control/energy swing up/energy injection ==
  x3 : Inport
  x4 : Inport  Port=2
  Cos : Trigonometry  Operator=cos
  Product : Product
  Sign : Signum
  minus_k_su : Gain  Gain=-k_su
  u_su : Outport
  wires:
  x3/1 -> Cos/1  "q"
  x4/1 -> Product/2  "q_d"
  Sign/1 -> minus_k_su/1
  minus_k_su/1 -> u_su/1
  Cos/1 -> Product/1
  Product/1 -> Sign/1

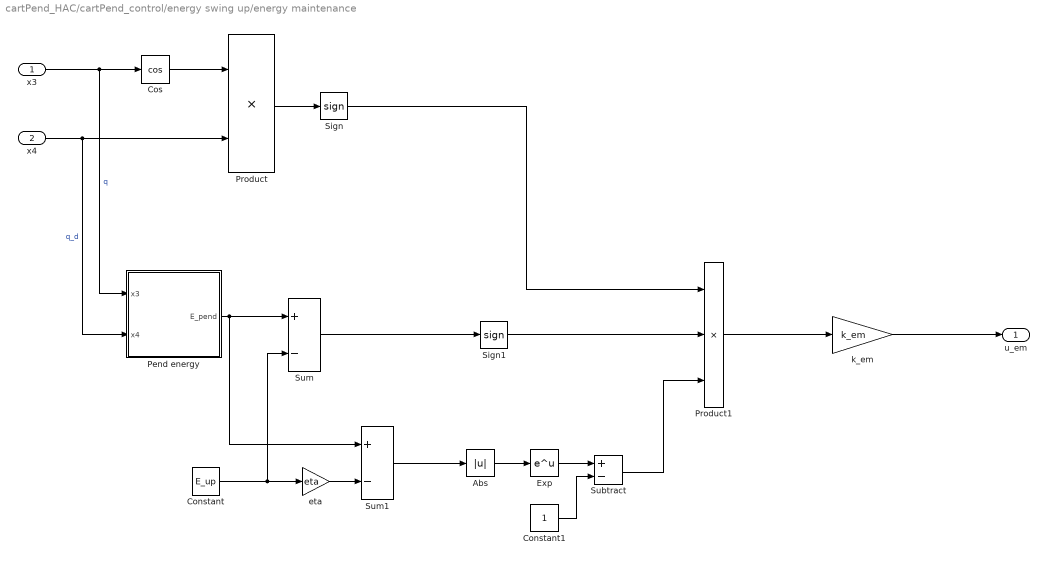
== system cartPend_HAC/cartPend_control/energy swing up/energy maintenance ==
  x3 : Inport
  x4 : Inport  Port=2
  Abs : Abs  SaturateOnIntegerOverflow=off
  Constant : Constant  Value=E_up
  Constant1 : Constant
  Cos : Trigonometry  Operator=cos
  Exp : Math
  Pend energy : Subsystem
  Product : Product
  Product1 : Product  Inputs=3
  Sign : Signum
  Sign1 : Signum
  Subtract : Sum  Inputs=+-
  Sum : Sum  Inputs=+-
  Sum1 : Sum  Inputs=+-
  eta : Gain  Gain=eta
  k_em : Gain  Gain=k_em
  u_em : Outport
  wires:
  x3/1 -> Pend energy/1(x3), Cos/1  "q"
  Cos/1 -> Product/1
  x4/1 -> Pend energy/2(x4), Product/2  "q_d"
  Product/1 -> Sign/1
  Pend energy/1(E_pend) -> Sum/1, Sum1/1
  Constant/1 -> Sum/2, eta/1
  Sum/1 -> Sign1/1
  eta/1 -> Sum1/2
  Sum1/1 -> Abs/1
  Abs/1 -> Exp/1
  Exp/1 -> Subtract/1
  Constant1/1 -> Subtract/2
  Sign1/1 -> Product1/2
  Sign/1 -> Product1/1
  Subtract/1 -> Product1/3
  Product1/1 -> k_em/1
  k_em/1 -> u_em/1

== system cartPend_HAC/cartPend_control/energy swing up/position potential well ==
  x1 : Inport
  Abs : Abs  SaturateOnIntegerOverflow=off
  Constant : Constant
  Gain1 : Gain  Gain=1/x1_max
  Log : Math  Operator=log
  Product : Product
  Sign : Signum
  Sum : Sum  Inputs=+-
  k_cw : Gain  Gain=k_cw
  u_cw : Outport
  wires:
  x1/1 -> Abs/1, Sign/1
  Abs/1 -> Gain1/1
  Gain1/1 -> Sum/2
  Constant/1 -> Sum/1
  Sum/1 -> Log/1
  k_cw/1 -> u_cw/1
  Product/1 -> k_cw/1
  Log/1 -> Product/2
  Sign/1 -> Product/1

== system cartPend_HAC/cartPend_control/energy swing up/velocity potential well ==
  x2 : Inport
  Abs : Abs  SaturateOnIntegerOverflow=off
  Constant : Constant
  Gain1 : Gain  Gain=1/x2_max
  Log : Math  Operator=log
  Product : Product
  Sign : Signum
  Sum : Sum  Inputs=+-
  k_vw : Gain  Gain=k_vw
  u_vw : Outport
  wires:
  Sign/1 -> Product/1
  Log/1 -> Product/2
  Product/1 -> k_vw/1
  k_vw/1 -> u_vw/1
  Sum/1 -> Log/1
  Constant/1 -> Sum/1
  Gain1/1 -> Sum/2
  Abs/1 -> Gain1/1
  x2/1 -> Sign/1, Abs/1

== system cartPend_HAC/HAC/HAC_thay_Le/Subsystem/If Action Subsystem3 ==
  Action Port : ActionPort  ActionPortLabel=if(u1 <= x_min)
  Constant : Constant  Value=u_min
  u_min : Outport
  wires:
  Constant/1 -> u_min/1

== system cartPend_HAC/HAC/HAC_thay_Le/Subsystem/If Action Subsystem4 ==
  Action Port : ActionPort  ActionPortLabel=elseif(u1 >= x_max)
  Constant : Constant  Value=u_max
  u_max : Outport
  wires:
  Constant/1 -> u_max/1

== system cartPend_HAC/HAC/HAC_thay_Le/Subsystem/If Action Subsystem5 ==
  x : Inport
  Action Port : ActionPort  ActionPortLabel=else
  Gain : Gain  Gain=u_max/x_max
  u_x : Outport
  wires:
  Gain/1 -> u_x/1
  x/1 -> Gain/1

== system cartPend_HAC/HAC/HAC_thay_Le/Subsystem1/If Action Subsystem3 ==
  Action Port : ActionPort  ActionPortLabel=if(u1 <= xd_min)
  Constant : Constant  Value=u_min
  u_min : Outport
  wires:
  Constant/1 -> u_min/1

== system cartPend_HAC/HAC/HAC_thay_Le/Subsystem1/If Action Subsystem4 ==
  Action Port : ActionPort  ActionPortLabel=elseif(u1 >= xd_max)
  Constant : Constant  Value=u_max
  u_max : Outport
  wires:
  Constant/1 -> u_max/1

== system cartPend_HAC/HAC/HAC_thay_Le/Subsystem1/If Action Subsystem5 ==
  xd : Inport
  Action Port : ActionPort  ActionPortLabel=else
  Gain : Gain  Gain=u_max/xd_max
  u_xd : Outport
  wires:
  xd/1 -> Gain/1
  Gain/1 -> u_xd/1

== system cartPend_HAC/HAC/HAC_thay_Le/Subsystem2/If Action Subsystem3 ==
  Action Port : ActionPort  ActionPortLabel=if(u1 <= q_min)
  Constant : Constant  Value=u_min
  u_min : Outport
  wires:
  Constant/1 -> u_min/1

== system cartPend_HAC/HAC/HAC_thay_Le/Subsystem2/If Action Subsystem4 ==
  Action Port : ActionPort  ActionPortLabel=elseif(u1 >= q_max)
  Constant : Constant  Value=u_max
  u_max : Outport
  wires:
  Constant/1 -> u_max/1

== system cartPend_HAC/HAC/HAC_thay_Le/Subsystem2/If Action Subsystem5 ==
  q : Inport
  Action Port : ActionPort  ActionPortLabel=else
  Gain : Gain  Gain=u_max/q_max
  u_q : Outport
  wires:
  Gain/1 -> u_q/1
  q/1 -> Gain/1

== system cartPend_HAC/HAC/HAC_thay_Le/Subsystem3/If Action Subsystem3 ==
  Action Port : ActionPort  ActionPortLabel=if(u1 <= qd_min)
  Constant : Constant  Value=u_min
  u_min : Outport
  wires:
  Constant/1 -> u_min/1

== system cartPend_HAC/HAC/HAC_thay_Le/Subsystem3/If Action Subsystem4 ==
  Action Port : ActionPort  ActionPortLabel=elseif(u1 >= qd_max)
  Constant : Constant  Value=u_max
  u_max : Outport
  wires:
  Constant/1 -> u_max/1

== system cartPend_HAC/HAC/HAC_thay_Le/Subsystem3/If Action Subsystem5 ==
  qd : Inport
  Action Port : ActionPort  ActionPortLabel=else
  Gain : Gain  Gain=u_max/qd_max
  u_qd : Outport
  wires:
  qd/1 -> Gain/1
  Gain/1 -> u_qd/1

== system cartPend_HAC/cartPend_control/HAC/HAC/If Action Subsystem ==
  Action Port : ActionPort  ActionPortLabel=if(u1 <= alpha)
  weight : Constant  Value=[0.25; 0.25; 0.25; 0.25]  VectorParams1D=off
  W : Outport
  wires:
  weight/1 -> W/1

== system cartPend_HAC/cartPend_control/HAC/HAC/If Action Subsystem1 ==
  Action Port : ActionPort  ActionPortLabel=elseif(u1 >= beta)
  weights : Constant  Value=[0; 0; 1; 0]  VectorParams1D=off
  W : Outport
  wires:
  weights/1 -> W/1

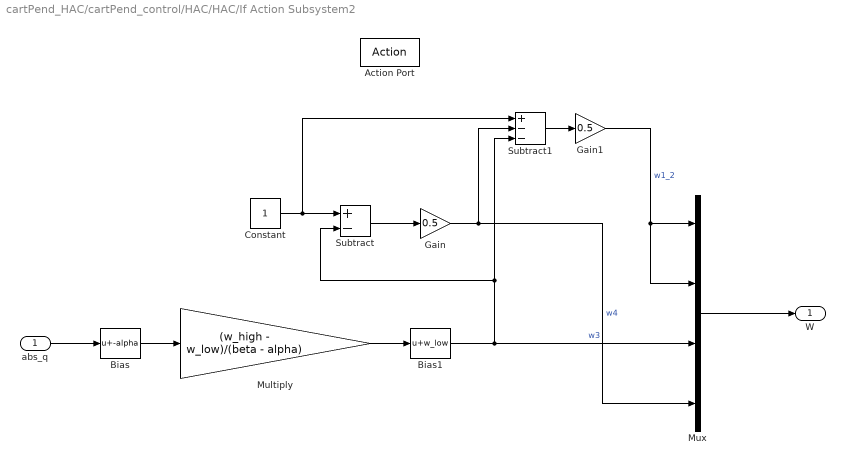
== system cartPend_HAC/cartPend_control/HAC/HAC/If Action Subsystem2 ==
  abs_q : Inport
  Action Port : ActionPort  ActionPortLabel=else
  Bias : Bias  Bias=-alpha  SaturateOnIntegerOverflow=off
  Bias1 : Bias  Bias=w_low  SaturateOnIntegerOverflow=off
  Constant : Constant
  Gain : Gain  Gain=0.5
  Gain1 : Gain  Gain=0.5
  Multiply : Gain  Gain=(w_high - w_low)/(beta - alpha)
  Mux : Mux
  Subtract : Sum  Inputs=+-
  Subtract1 : Sum  Inputs=+--
  W : Outport
  wires:
  Mux/1 -> W/1
  abs_q/1 -> Bias/1
  Bias/1 -> Multiply/1
  Multiply/1 -> Bias1/1
  Bias1/1 -> Subtract/2, Subtract1/3, Mux/3  "w3"
  Constant/1 -> Subtract1/1, Subtract/1
  Subtract/1 -> Gain/1
  Gain/1 -> Subtract1/2, Mux/4  "w4"
  Subtract1/1 -> Gain1/1
  Gain1/1 -> Mux/1, Mux/2  "w1_2"

== system cartPend_HAC/cartPend_control/HAC/HAC/denorm_u ==
  U_s : Inport
  Bias : Bias  Bias=u_min  SaturateOnIntegerOverflow=off
  Gain : Gain  Gain=u_max - u_min
  U : Outport
  wires:
  U_s/1 -> Gain/1
  Gain/1 -> Bias/1
  Bias/1 -> U/1

== system cartPend_HAC/cartPend_control/HAC/HAC/denorm_u1 ==
  U_s : Inport
  Bias : Bias  Bias=u_min  SaturateOnIntegerOverflow=off
  Gain : Gain  Gain=u_max - u_min
  U : Outport
  wires:
  Bias/1 -> U/1
  Gain/1 -> Bias/1
  U_s/1 -> Gain/1

== system cartPend_HAC/cartPend_control/HAC/HAC/denorm_u2 ==
  U_s : Inport
  Bias : Bias  Bias=u_min  SaturateOnIntegerOverflow=off
  Gain : Gain  Gain=u_max - u_min
  U : Outport
  wires:
  U_s/1 -> Gain/1
  Gain/1 -> Bias/1
  Bias/1 -> U/1

== system cartPend_HAC/cartPend_control/HAC/HAC/denorm_u3 ==
  U_s : Inport
  Bias : Bias  Bias=u_min  SaturateOnIntegerOverflow=off
  Gain : Gain  Gain=u_max - u_min
  U : Outport
  wires:
  Bias/1 -> U/1
  Gain/1 -> Bias/1
  U_s/1 -> Gain/1

== system cartPend_HAC/cartPend_control/HAC/HAC_thay_Le/If Action Subsystem ==
  Action Port : ActionPort  ActionPortLabel=if(u1 <= alpha)
  weight : Constant  Value=[0.25; 0.25; 0.25; 0.25]  VectorParams1D=off
  W : Outport
  wires:
  weight/1 -> W/1

== system cartPend_HAC/cartPend_control/HAC/HAC_thay_Le/If Action Subsystem1 ==
  Action Port : ActionPort  ActionPortLabel=elseif(u1 >= beta)
  weights : Constant  Value=[0; 0; 1; 0]  VectorParams1D=off
  W : Outport
  wires:
  weights/1 -> W/1

== system cartPend_HAC/cartPend_control/HAC/HAC_thay_Le/If Action Subsystem2 ==
  abs_q : Inport
  Action Port : ActionPort  ActionPortLabel=else
  Bias : Bias  Bias=-alpha  SaturateOnIntegerOverflow=off
  Bias1 : Bias  Bias=w_low  SaturateOnIntegerOverflow=off
  Constant : Constant
  Gain : Gain  Gain=0.5
  Gain1 : Gain  Gain=0.5
  Multiply : Gain  Gain=(w_high - w_low)/(beta - alpha)
  Mux : Mux
  Subtract : Sum  Inputs=+-
  Subtract1 : Sum  Inputs=+--
  W : Outport
  wires:
  Gain1/1 -> Mux/4, Mux/2  "w2_4"
  Subtract1/1 -> Gain1/1
  Gain/1 -> Mux/1, Subtract1/2  "w1"
  Subtract/1 -> Gain/1
  Constant/1 -> Subtract/1, Subtract1/1
  Bias1/1 -> Mux/3, Subtract1/3, Subtract/2  "w3"
  Multiply/1 -> Bias1/1
  Bias/1 -> Multiply/1
  abs_q/1 -> Bias/1
  Mux/1 -> W/1

== system cartPend_HAC/cartPend_control/HAC/HAC_thay_Le/denorm_u3 ==
  U_s : Inport
  Bias : Bias  Bias=u_min  SaturateOnIntegerOverflow=off
  Gain : Gain  Gain=u_max - u_min
  U : Outport
  wires:
  U_s/1 -> Gain/1
  Gain/1 -> Bias/1
  Bias/1 -> U/1

== system cartPend_HAC/cartPend_control/energy swing up/energy maintenance/Pend energy ==
  x3 : Inport
  x4 : Inport  Port=2
  Cos : Trigonometry  Operator=cos
  Gain : Gain  Gain=m*g*L
  Gain1 : Gain  Gain=0.5*(I+m*L^2)
  Square : Math  Operator=square
  Sum : Sum
  E_pend : Outport
  wires:
  x3/1 -> Cos/1  "q"
  x4/1 -> Square/1  "q_d"
  Cos/1 -> Gain/1
  Square/1 -> Gain1/1
  Gain/1 -> Sum/1
  Gain1/1 -> Sum/2
  Sum/1 -> E_pend/1
